simulink model "adcs_visual_20230921"  (R2023b)
settings: Solver=ode45  StartTime=0.0  StopTime=100000  RelTol=1e-3
InitFcn:
  | % Define the parameters
  | core_radius = 0.005;
  | core_length = 0.045;
  | layers = 6;
  | temp = 20;
  | side_length = 0.045;
  | air_length = 0.025;
  | air_layers = 5;
  | 
  | coreMagX = CoreMagnetorquer(core_radius, core_length, layers, temp);
  | coreMagY = CoreMagnetorquer(core_radius, core_length, layers, temp);
  | airMagZ = AirMagnetorquer(side_length, air_length, air_layers, temp);
libraries: shared6dof x1, simulink x1
settings Model: Creator=steve  LastModifiedBy=bobow

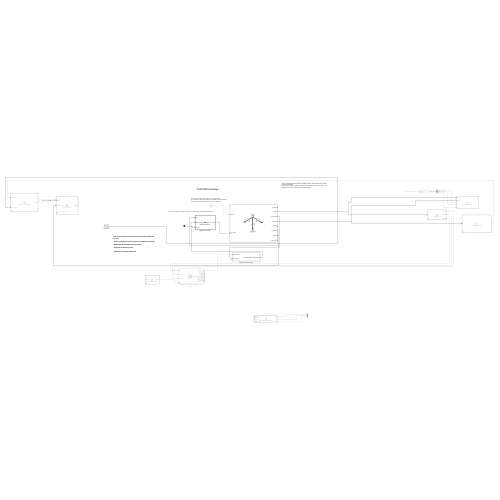
[thumbnail: Simulink's stored preview of the top-level diagram]
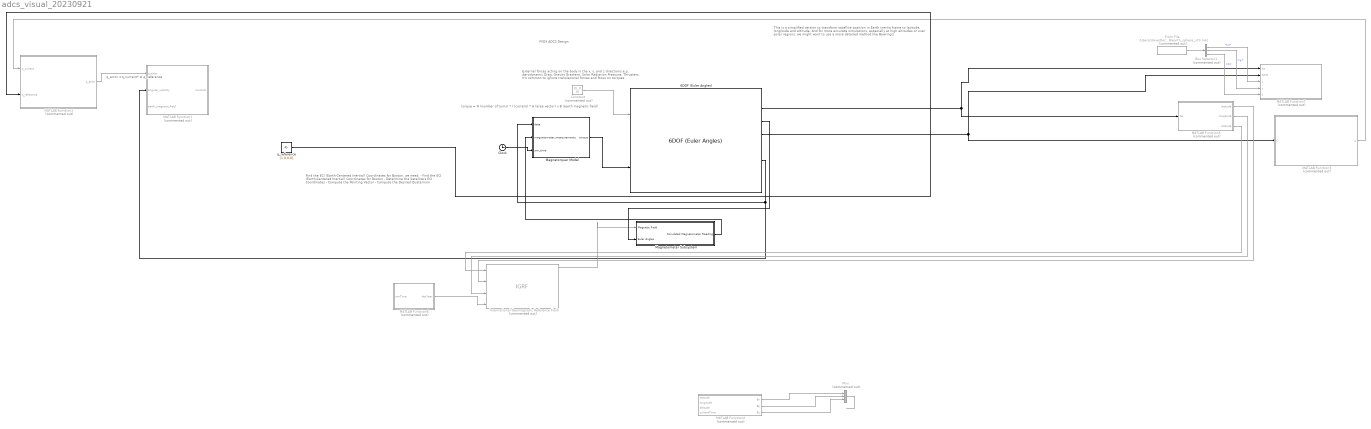
== system adcs_visual_20230921 ==
  note: torque = N (number of turns) * I (current) * A (area vector) x B (earth magnetic field)
  note: q_error =q_current* ⊗ q_reference
      | ​
  note: This is a simplified version to transform satellite position in Earth inertia frame to latitude, longitude and altitude,
      | And for more accurate simulations, especially at high altitudes or over polar regions, we might want to use a more detailed method like Bowring's
  note: PVDX ADCS Design
  note: Find the ECI (Earth-Centered Inertial) Coordinates for Boston, we need:
      | - Find the ECI (Earth-Centered Inertial) Coordinates for Boston
      | - Determine the Satellite's ECI Coordinates
      | - Compute the Pointing Vector
      | - Compute the Desired Quaternion
  note: External forces acting on the body in the x, y, and z directions
      | e.g. Aerodynamic Drag, Gravity Gradient, Solar Radiation Pressure, Thrusters.
      | It's common to ignore translational forces and focus on torques
  6DOF (Euler Angles) : shared6dof/6DOF (Euler Angles)  units=Metric (MKS)  mtype=Fixed  rep=Quaternion  xme_0=[0 0 0]  Vm_0=[0 0 0]  eul_0=[0 -3.1415926/2 0]  pm_0=-[0.1 0.1 0.1]  mass_0=3.0  mass_e=0.5  mass_f=2.0  inertia=eye(3)  inertia_e=eye(3)  inertia_f=2*eye(3)  k_quat=1.0  vre_flag=on  abi_flag=off  aMode=0  xme_statename=''  Vm_statename=''  eul_statename=''  quat_statename=''  pm_statename=''  mass_statename=''
  Bus Selector1 : BusSelector  Commented=on  OutputSignals=x,y,z
  Clock : Clock
  Constant : Constant  Commented=on  Value=[0, 0, 0]
  From File : FromFile  Commented=on  FileName=/Users/steve/Documents/Brown/BSE/ADCS/ADCS_Visual_MATLAB/earth_sphere_v73.mat  OutDataTypeStr=Bus: SphereBus  SampleTime=0
  International Geomagnetic Reference Field : IGRF  Commented=on  month=January  day=1  year=2020
      settings: AttributesFormatString=%<generation>
  MATLAB Function1 : MATLAB Function  Commented=on  TreatAsAtomicUnit=on
  MATLAB Function2 : MATLAB Function  Commented=on  TreatAsAtomicUnit=on
  MATLAB Function3 : MATLAB Function  Commented=on  TreatAsAtomicUnit=on
  MATLAB Function4 : MATLAB Function  Commented=on  TreatAsAtomicUnit=on
  MATLAB Function5 : MATLAB Function  Commented=on  TreatAsAtomicUnit=on
  MATLAB Function6 : MATLAB Function  Commented=on  TreatAsAtomicUnit=on
  MATLAB Function7 : MATLAB Function  Commented=on  TreatAsAtomicUnit=on  SystemSampleTime=0.1
  Magnetometer Subsystem : Subsystem
  Magnetorquer Model : MATLAB Function  TreatAsAtomicUnit=on  SystemSampleTime=0
  Mux : Mux  Commented=on  Inputs=3
  q_reference : Constant  Value=[1,0,0,0]  VectorParams1D=off
  wires:
  Magnetorquer Model/1(torque) -> 6DOF (Euler Angles)/2
  Constant/1 -> 6DOF (Euler Angles)/1
  6DOF (Euler Angles)/6 -> MATLAB Function1/2(angular_velocity), Magnetorquer Model/1(data)
  6DOF (Euler Angles)/4 -> MATLAB Function7/2(DCM), MATLAB Function3/1(C)
  MATLAB Function3/1(q) -> MATLAB Function2/1(q_current)
  q_reference/1 -> MATLAB Function2/2(q_reference)
  MATLAB Function4/1(Bx) -> Mux/1
  MATLAB Function4/2(By) -> Mux/2
  MATLAB Function4/3(Bz) -> Mux/3
  Mux/1 -> ?
  6DOF (Euler Angles)/2 -> MATLAB Function7/1(Xe), MATLAB Function5/1(Xe)
  MATLAB Function5/1(latitude) -> International Geomagnetic Reference Field/2
  MATLAB Function5/2(longitude) -> International Geomagnetic Reference Field/3
  MATLAB Function5/3(altitude) -> International Geomagnetic Reference Field/1
  Clock/1 -> Magnetorquer Model/3(sim_time)
  MATLAB Function6/1(decYear) -> International Geomagnetic Reference Field/4
  Magnetometer Subsystem/1(Simulated Magnetometer Reading) -> Magnetorquer Model/2(magnetometer_measurements)
  MATLAB Function2/1(q_error) -> MATLAB Function1/1(q_error)
  From File/1 -> Bus Selector1/1
  Bus Selector1/1 -> MATLAB Function7/3(x)  "<x>"
  Bus Selector1/2 -> MATLAB Function7/4(y)  "<y>"
  Bus Selector1/3 -> MATLAB Function7/5(z)  "<z>"
  International Geomagnetic Reference Field/1 -> Magnetometer Subsystem/1(Magnetic Field)
  6DOF (Euler Angles)/3 -> Magnetometer Subsystem/2(Euler Angles)

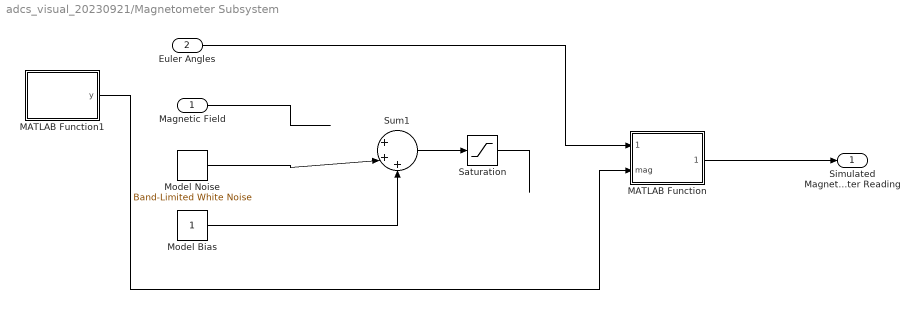
== system adcs_visual_20230921/Magnetometer Subsystem ==
  Magnetic Field : Inport  PortDimensions=3
  Euler Angles : Inport  Port=2
  MATLAB Function : MATLAB Function  TreatAsAtomicUnit=on  SystemSampleTime=0
  MATLAB Function1 : MATLAB Function  TreatAsAtomicUnit=on  SystemSampleTime=0
  Model Bias : Constant
  Model Noise : simulink/Sources/Band-Limited White Noise  Cov=[0.1]  Ts=0.1  seed=[23341]
  Saturation : Saturate
  Sum1 : Sum  Inputs=|+++
  Simulated Magnetometer Reading : Outport  SampleTime=0
  wires:
  Magnetic Field/1 -> ?
  Model Noise/1 -> Sum1/2
  Model Bias/1 -> Sum1/3
  Sum1/1 -> Saturation/1
  Saturation/1 -> ?
  Euler Angles/1 -> MATLAB Function/1(euler_angles)
  MATLAB Function/1(reading) -> Simulated Magnetometer Reading/1
  MATLAB Function1/1(y) -> MATLAB Function/2(mag)

== matlab function adcs_visual_20230921/MATLAB Function1 ==
  data: q_error input; currents output; angular_velocity input; earth_magnetic_field input
function currents = controlAlgorithm(q_error, angular_velocity, earth_magnetic_field)
    % Ensure inputs are column vectors
    q_error_vec = q_error(2:4).';  % Extract the vector part of the quaternion
    angular_velocity = angular_velocity(:);
    earth_magnetic_field = earth_magnetic_field(:);

    % Proportional and Derivative control gains
    Kp = diag([1, 1, 1]);  % Proportional gain matrix
    Kd = diag([0.5, 0.5, 0.5]);  % Derivative gain matrix

    % PD Controller using the vector part of the quaternion error
    desired_torque = -Kp * q_error_vec - Kd * angular_velocity;

    % Compute the required magnetic moment for the desired torque.
    % Assuming the torque is the cross product of the magnetic moment and the Earth's magnetic field: 
    % torque = m x B => m = torque x B (for simplicity; this is an approximation).
    desired_magnetic_moment = cross(desired_torque, earth_magnetic_field);

    % Magnetorquer properties
    N = 100;  % Number of turns in the coil (example value)
    A = 0.01 * 0.01;  % Area of the coil, 1cm x 1cm (example value)

    % Convert desired magnetic moment to required current for each magnetorquer
    currents = desired_magnetic_moment ./ (N * A);
    
    % Safety check
    if currents(1) > 0.1
        currents(1) = 0.1;
    end
    if currents(2) > 0.1
        currents(2) = 0.1;
    end
    if currents(3) > 0.1
        currents(3) = 0.1;
    end

end

== matlab function adcs_visual_20230921/Magnetorquer Model ==
  settings: updateMethod=DISCRETE
  data: data input; magnetometer_measurements input; torque output; sim_time input
function torque = magnetorquerModel(data, magnetometer_measurements, sim_time)
    persistent coreMagX coreMagY airMagZ prev_measurement prev_time
    data
    % Define the parameters
    core_radius = 0.005;
    core_length = 0.045;
    layers = 6;
    temp = 20;
    side_length = 0.045;
    air_length = 0.025;
    air_layers = 5;

    if isempty(coreMagX) || isempty(coreMagY) || isempty(airMagZ)
        coreMagX = CoreMagnetorquer(core_radius, core_length, layers, temp);
        coreMagY = CoreMagnetorquer(core_radius, core_length, layers, temp);  
        airMagZ = AirMagnetorquer(side_length, air_length, air_layers, temp);
    end

    if isempty(prev_measurement) || isempty(prev_time)
        prev_measurement = magnetometer_measurements;
        prev_time = sim_time;
    end

    b_dot = (magnetometer_measurements - prev_measurement);
    
    % currents = -[coreMagX.calc_current(b_dot(1)),...
    %     coreMagY.calc_current(b_dot(2)),...
    %     airMagZ.calc_current(b_dot(3))];
    % 
    % 
    % m  = [coreMagX.calc_dipole_moment(currents(1))...
    %     coreMagY.calc_dipole_moment(currents(2))...
    %     airMagZ.calc_dipole_moment(currents(3))];

    k = 1;

    m = -k*b_dot/(norm(b_dot)+1e-16)
    if abs(m(1)) > coreMagX.max_dipole
        disp('1 saturated')
        m(1) = coreMagX.max_dipole * sign(m(1))
    end
    if abs(m(2)) > coreMagY.max_dipole
        disp('2 saturated')
        m(2) = coreMagY.max_dipole * sign(m(2))
    end
    if abs(m(3)) > airMagZ.max_dipole
        disp('3 saturated')
        m(3) = airMagZ.max_dipole * sign(m(3))
    end
    prev_measurement = magnetometer_measurements;
    prev_time = sim_time;
    
    % Torque = m x B
    torque = cross(m, magnetometer_measurements)
end

== matlab function adcs_visual_20230921/MATLAB Function2 ==
  data: q_current input; q_error output; q_reference input
function q_error = computeAttitudeError(q_current, q_reference)
    % Compute the conjugate of the current quaternion
    q_current_star = [q_current(1), -q_current(2:4)];
    
    % Multiply the conjugate of the current quaternion with the reference quaternion
    q_error = quatmultiply(q_current_star, q_reference);
end

== matlab function adcs_visual_20230921/MATLAB Function3 ==
  data: C input; q output
function q = DCMtoQuaternion(C)
    % Extract individual elements from the DCM
    C11 = C(1,1);
    C12 = C(1,2);
    C13 = C(1,3);
    C21 = C(2,1);
    C22 = C(2,2);
    C23 = C(2,3);
    C31 = C(3,1);
    C32 = C(3,2);
    C33 = C(3,3);

    % Compute quaternion components
    q0 = 0.5 * sqrt(1 + C11 + C22 + C33);
    q1 = (1/(4*q0)) * (C32 - C23);
    q2 = (1/(4*q0)) * (C13 - C31);
    q3 = (1/(4*q0)) * (C21 - C12);

    % Compile quaternion and normalize
    q = [q0, q1, q2, q3];
    q = q / norm(q);
end

== matlab function adcs_visual_20230921/MATLAB Function4 ==
  data: latitude input; Bx output; longitude input; altitude input; currentTime input; By output; Bz output
function [Bx, By, Bz] = geomagneticFieldModel(latitude, longitude, altitude, currentTime)
    % Convert latitude and longitude from degrees to radians
    % latRad = deg2rad(latitude);
    % lonRad = deg2rad(longitude);

    [XYZ,~,~,~,~] ...
        = igrfmagm(altitude, latitude, longitude, currentTime);
    [Bx, By, Bz] = deal(XYZ);
    % magFieldVector = igrf11magm(altitude, latRad, lonRad, currentTime);
    % Bx = magFieldVector(1);
    % Bx = 0;
    % By = magFieldVector(2);
    % By = 45e-6;
    % Bz = magFieldVector(3);
    % Bz = 0;
    % The outputs Bx, By, and Bz represent the magnetic field components in nanoTesla (nT).
end

== matlab function adcs_visual_20230921/MATLAB Function5 ==
  data: Xe input; latitude output; longitude output; altitude output
function [latitude, longitude, altitude] = ECEFtoLLA(Xe)
    % Earth's constants (WGS-84 ellipsoidal parameters)
    a = 6378137;         % Equatorial radius (meters)
    f = 1/298.257223563; % Flattening factor
    b = (1-f)*a;         % Polar radius

    % Extract the coordinates
    x = Xe(1);
    y = Xe(2);
    z = Xe(3);

    % Longitude
    longitude = atan2(y, x);

    % Simplified Latitude and Altitude (spherical Earth)
    rho = sqrt(x^2 + y^2);
    latitude = atan2(z, rho);
    altitude = rho / cos(latitude) - a;

    % Note: For more accurate conversions, consider implementing
    % a method like Bowring's to account for the Earth's oblateness.
end

== matlab function adcs_visual_20230921/MATLAB Function6 ==
  data: simTime input; decYear output
function decYear = simTimeToDecimalYear(simTime)

    % Define the epoch (starting date) - e.g., 1st Jan 2023
    epochYear = 2023;
    secondsInYear = 365 * 24 * 60 * 60; % Assuming non-leap year for simplicity
    
    % Compute elapsed years and remaining seconds since the epoch
    elapsedYears = floor(simTime / secondsInYear);
    remainingSeconds = mod(simTime, secondsInYear);

    % Determine the current year
    currentYear = epochYear + elapsedYears;

    % Check if the current year is a leap year
    isLeapYear = mod(currentYear, 4) == 0 & (mod(currentYear, 100) ~= 0 | mod(currentYear, 400) == 0);
    
    if isLeapYear
        secondsInYear = 366 * 24 * 60 * 60; % Adjust for leap year
    end

    % Compute the fraction of the year
    yearFraction = remainingSeconds / secondsInYear;

    % Compute the decimal year
    decYear = currentYear + yearFraction;

end

== matlab function adcs_visual_20230921/MATLAB Function7 ==
  data: Xe input; DCM input; x input; y input; z input
function visualizeSatellite(Xe, DCM, x, y, z)
    % Extract direction from DCM
    dirX = DCM(:, 1);
    dirY = DCM(:, 2);
    dirZ = DCM(:, 3);

    % Maintain history of the positions
    persistent historyX historyY historyZ;
    if isempty(historyX)
        historyX = [];
        historyY = [];
        historyZ = [];
    end

    historyX(end+1) = Xe(1);
    historyY(end+1) = Xe(2);
    historyZ(end+1) = Xe(3);

    % Earth plot (simple sphere representation)
    surf(x*6371, y*6371, z*6371, 'FaceColor', [0 0 1], 'FaceAlpha', 0.5); % Earth radius ~6371 km
    hold on;

    % Plot the trajectory
    plot3(historyX, historyY, historyZ, 'r-', 'LineWidth', 1.5);

    % Represent the body axes
    quiver3(Xe(1), Xe(2), Xe(3), dirX(1), dirX(2), dirX(3), 'r', 'LineWidth', 2);
    quiver3(Xe(1), Xe(2), Xe(3), dirY(1), dirY(2), dirY(3), 'g', 'LineWidth', 2);
    quiver3(Xe(1), Xe(2), Xe(3), dirZ(1), dirZ(2), dirZ(3), 'b', 'LineWidth', 2);

    surface_point = (Xe / norm(Xe)) * 6371; % Point on Earth's surface directly below the satellite
    plot3([surface_point(1), Xe(1)], [surface_point(2), Xe(2)], [surface_point(3), Xe(3)], 'k--');

    altitude = norm(Xe) - 6371; % Subtract Earth's radius
    
    % Check if the current position is the latest position
    if length(historyX) == numel(Xe(1))
        text(Xe(1), Xe(2), Xe(3), sprintf('Altitude: %.2f km', altitude));
    end

    % Define vertices for the satellite body (10x10x30 cm)
    vertices = [0 0 0; 0 10 0; 10 10 0; 10 0 0; 0 0 30; 0 10 30; 10 10 30; 10 0 30];
    vertices = vertices + repmat(Xe', 8, 1); % Adjust vertices based on Xe
    faces = [1 2 3 4; 5 6 7 8; 1 2 6 5; 2 3 7 6; 3 4 8 7; 4 1 5 8];
    patch('Vertices', vertices, 'Faces', faces, 'FaceColor', 'blue');

    % Camera and view settings to keep Earth centered
    rotate3d on;  % enable 3D rotation
    axis equal;
    xlabel('X (m)');
    ylabel('Y (m)');
    zlabel('Z (m)');
    grid on;
    drawnow; % Update the plot
    view(3); % This sets the axes to a 3D perspective.
end

== matlab function adcs_visual_20230921/Magnetometer Subsystem/MATLAB Function ==
  settings: updateMethod=DISCRETE
  data: euler_angles input; reading output; mag input
function reading = fcn(euler_angles, mag)
    persistent Rz_yaw Ry_pitch Rx_roll R
    
    roll = euler_angles(1);
    pitch = euler_angles(2);
    yaw = euler_angles(3);

    Rz_yaw = [cos(yaw) -sin(yaw) 0; sin(yaw) cos(yaw) 0; 0 0 1];
    Ry_pitch = [cos(pitch) 0 sin(pitch); 0 1 0; -sin(pitch) 0 cos(pitch)];
    Rx_roll = [1 0 0; 0 cos(roll) -sin(roll); 0 sin(roll) cos(roll)];
    
    % Compute the final rotation matrix
    R = Rz_yaw * Ry_pitch * Rx_roll;
    
    reading = R * mag;

== matlab function adcs_visual_20230921/Magnetometer Subsystem/MATLAB Function1 ==
  data: y output
function y = fcn()

y =    1.0e-05 * [2.1439; 0.1641; 3.8676];
